simulink model "exercise_05_05_i_pd_cont"  (R2018b)
settings: Solver=ode4  StartTime=0.0  StopTime=1  FixedStep=0.001  RelTol=1e-3
undefined symbols (not defined in the file): c, dc, kD, kI, kP, M, rc
settings Model: Creator=kawata  LastModifiedBy=kawata

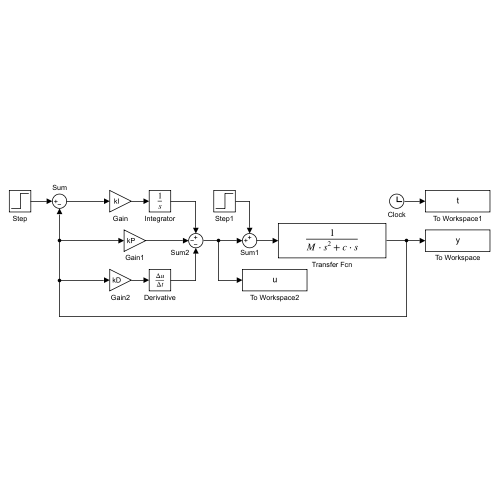
[thumbnail: Simulink's stored preview of the top-level diagram]
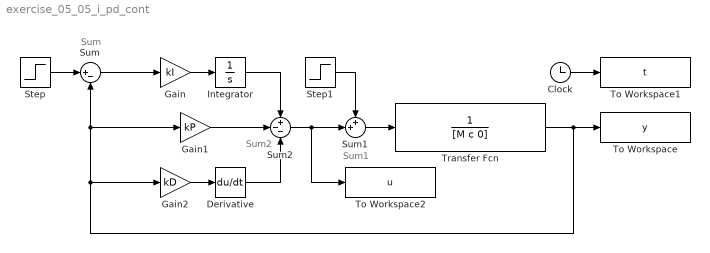
== system exercise_05_05_i_pd_cont ==
  note: Sum
  note: Sum1
  note: Sum2
  Clock : Clock
  Derivative : Derivative
  Gain : Gain  Gain=kI
  Gain1 : Gain  Gain=kP
  Gain2 : Gain  Gain=kD
  Integrator : Integrator
  Step : Step  Time=0  After=rc  SampleTime=0
  Step1 : Step  Time=1.5  After=dc  SampleTime=0
  Sum : Sum  Inputs=|+-
  Sum1 : Sum  Inputs=++|
  Sum2 : Sum  Inputs=+--
  To Workspace : ToWorkspace  VariableName=y  SampleTime=-1
  To Workspace1 : ToWorkspace  VariableName=t  SampleTime=-1
  To Workspace2 : ToWorkspace  VariableName=u  SampleTime=-1
  Transfer Fcn : TransferFcn  Denominator=[M c 0]
  wires:
  Step1/1 -> Sum1/1
  Sum2/1 -> To Workspace2/1, Sum1/2
  Sum1/1 -> Transfer Fcn/1
  Integrator/1 -> Sum2/1
  Gain1/1 -> Sum2/2
  Derivative/1 -> Sum2/3
  Gain2/1 -> Derivative/1
  Sum/1 -> Gain/1
  Gain/1 -> Integrator/1
  Step/1 -> Sum/1
  Transfer Fcn/1 -> To Workspace/1, Gain2/1, Gain1/1, Sum/2
  Clock/1 -> To Workspace1/1
